simulink model "lab3"  (R2017b)
settings: Solver=VariableStepAuto  StartTime=0.0  StopTime=3.5  RelTol=1e-3
settings Model: Creator=ayushi  LastModifiedBy=ayushi

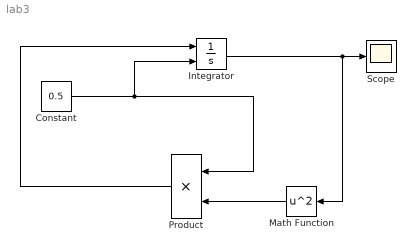
== system lab3 ==
  Constant : Constant  Value=0.5
  Integrator : Integrator  InitialConditionSource=external
  Math Function : Math  Operator=square  SaturateOnIntegerOverflow=on
  Product : Product
  Scope : Scope
  wires:
  Constant/1 -> Product/1, Integrator/2
  Product/1 -> Integrator/1
  Math Function/1 -> Product/2
  Integrator/1 -> Math Function/1, Scope/1
